simulink model "doubleloop"  (R2022a)
settings: Solver=VariableStepAuto  StartTime=0.0  StopTime=10.0  RelTol=1e-3
undefined symbols (not defined in the file): AS, BS, CS, DS
settings Model: Creator=jeffr  LastModifiedBy=jeffr

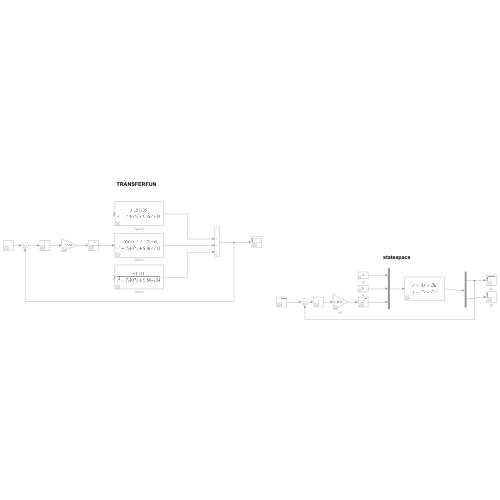
[thumbnail: Simulink's stored preview of the top-level diagram]
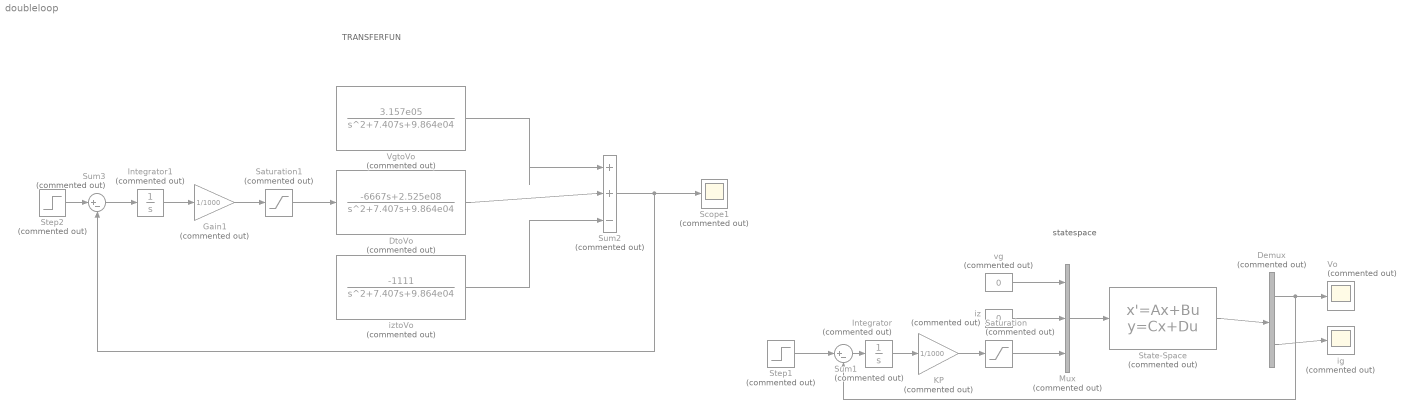
== system doubleloop ==
  note: TRANSFERFUN
  note: statespace
  Demux : Demux  Commented=on  Outputs=2
  DtoVo : TransferFcn  Commented=on  Numerator="[-6667  2.525e08]"  Denominator="[1 7.407  9.864e04]"
  Gain1 : Gain  Commented=on  Gain=1/1000
  Integrator : Integrator  Commented=on
  Integrator1 : Integrator  Commented=on
  KP : Gain  Commented=on  Gain=1/1000
  Mux : Mux  Commented=on  Inputs=3
  Saturation : Saturate  Commented=on
  Saturation1 : Saturate  Commented=on  UpperLimit=1  LowerLimit=0
  Scope1 : Scope  Commented=on
  State-Space : StateSpace  Commented=on  A=AS  B=BS  C=CS  D=DS  InitialCondition=0
  Step1 : Step  Commented=on  Time=5  Before=1  After=800  SampleTime=0
  Step2 : Step  Commented=on  Time=5  Before=800  After=800  SampleTime=0
  Sum1 : Sum  Commented=on  Inputs=|+-
  Sum2 : Sum  Commented=on  Inputs=|++-
  Sum3 : Sum  Commented=on  Inputs=|+-
  VgtoVo : TransferFcn  Commented=on  Numerator=[3.157e05]  Denominator="[1 7.407  9.864e04]"
  Vo : Scope  Commented=on
  ig : Scope  Commented=on
  iz : Constant  Commented=on  Value=0
  iztoVo : TransferFcn  Commented=on  Numerator=[-1111]  Denominator="[1 7.407  9.864e04]"
  vg : Constant  Commented=on  Value=0
  wires:
  iz/1 -> Mux/2
  Integrator1/1 -> Gain1/1
  Step2/1 -> Sum3/1
  Gain1/1 -> Saturation1/1
  Saturation1/1 -> DtoVo/1
  Sum3/1 -> Integrator1/1
  Integrator/1 -> KP/1
  Sum2/1 -> Scope1/1, Sum3/2
  Step1/1 -> Sum1/1
  Sum1/1 -> Integrator/1
  VgtoVo/1 -> Sum2/1
  Demux/1 -> Vo/1, Sum1/2
  Saturation/1 -> Mux/3
  KP/1 -> Saturation/1
  Demux/2 -> ig/1
  State-Space/1 -> Demux/1
  Mux/1 -> State-Space/1
  DtoVo/1 -> Sum2/2
  vg/1 -> Mux/1
  iztoVo/1 -> Sum2/3
